simulink model "tankcontrol_linearised_model_PI_controller_control101"  (R2025b)
settings: Solver=VariableStepAuto  StartTime=0.0  StopTime=300  RelTol=1e-3
undefined symbols (not defined in the file or in its folder): alfa1rel, alfa2rel, beta1rel, delta2rel, h10rel, h20rel, u0
settings Model: Creator=barsr  LastModifiedBy=barsr
settings RTWCC: GPUComputeCapability=3.5

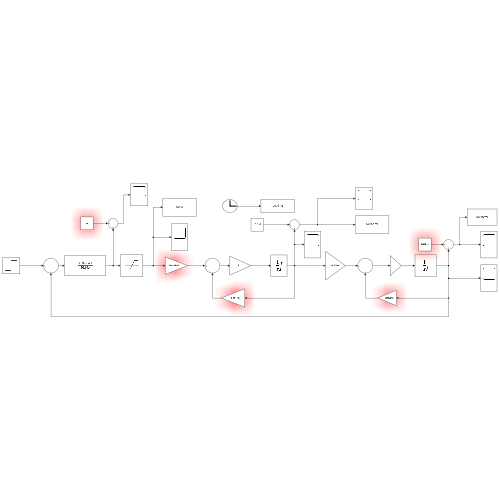
[thumbnail: Simulink's stored preview of the top-level diagram]
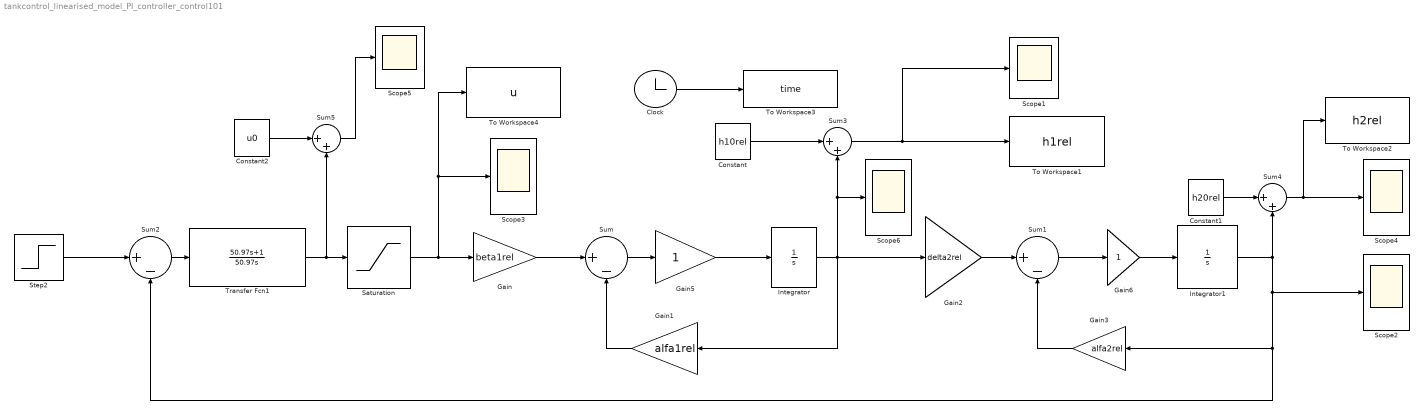
== system tankcontrol_linearised_model_PI_controller_control101 ==
  Clock : Clock
  Constant : Constant  Value=h10rel
  Constant1 : Constant  Value=h20rel
  Constant2 : Constant  Value=u0
  Gain : Gain  Gain=beta1rel
  Gain1 : Gain  Gain=alfa1rel
  Gain2 : Gain  Gain=delta2rel
  Gain3 : Gain  Gain=alfa2rel
  Gain5 : Gain
  Gain6 : Gain
  Integrator : Integrator  LimitOutput=on  UpperSaturationLimit=1  LowerSaturationLimit=0
  Integrator1 : Integrator  LimitOutput=on  UpperSaturationLimit=1  LowerSaturationLimit=0
  Saturation : Saturate  UpperLimit=1  LowerLimit=0
  Scope{1..6} (6 alike) : Scope
      Scope1 settings: ActiveDisplayYMinimum=0.047933990579917485  ActiveDisplayYMaximum=0.4377411736304716
      Scope2 settings: ActiveDisplayYMinimum=-0.76866162703230412  ActiveDisplayYMaximum=1.4291405570926656
      Scope3 settings: ActiveDisplayYMinimum=-0.82951581487383041  ActiveDisplayYMaximum=2.9648640057466338
      Scope4 settings: ActiveDisplayYMinimum=-0.76866162703230412  ActiveDisplayYMaximum=1.4291405570926656  DataLoggingVariableName=ScopeData2
      Scope5 settings: ActiveDisplayYMinimum=-0.28268319394776326  ActiveDisplayYMaximum=0.65543427021264211  DataLoggingVariableName=ScopeData3
      Scope6 settings: ActiveDisplayYMinimum=-0.76866162703230412  ActiveDisplayYMaximum=1.4291405570926656  DataLoggingVariableName=ScopeData4
  Step2 : Step  Time=0  After=0.3  SampleTime=0
  Sum : Sum  Inputs=|+-
  Sum1 : Sum  Inputs=|+-
  Sum2 : Sum  Inputs=|+-
  Sum3 : Sum  Inputs=|++
  Sum4 : Sum  Inputs=|++
  Sum5 : Sum  Inputs=|++
  To Workspace1 : ToWorkspace  VariableName=h1rel  SampleTime=-1
  To Workspace2 : ToWorkspace  VariableName=h2rel  SampleTime=-1
  To Workspace3 : ToWorkspace  VariableName=time  SampleTime=-1
  To Workspace4 : ToWorkspace  VariableName=u  SampleTime=-1
  Transfer Fcn1 : TransferFcn  Numerator=[50.97 1]  Denominator=[50.97 0]
  wires:
  Gain/1 -> Sum/1
  Sum/1 -> Gain5/1
  Integrator/1 -> Gain2/1, Gain1/1, Scope6/1, Sum3/2
  Sum1/1 -> Gain6/1
  Gain5/1 -> Integrator/1
  Gain6/1 -> Integrator1/1
  Gain1/1 -> Sum/2
  Gain3/1 -> Sum1/2
  Clock/1 -> To Workspace3/1
  Step2/1 -> Sum2/1
  Sum2/1 -> Transfer Fcn1/1
  Saturation/1 -> To Workspace4/1, Scope3/1, Gain/1
  Constant/1 -> Sum3/1
  Sum3/1 -> Scope1/1, To Workspace1/1
  Constant1/1 -> Sum4/1
  Gain2/1 -> Sum1/1
  Sum4/1 -> To Workspace2/1, Scope4/1
  Integrator1/1 -> Sum4/2, Scope2/1, Gain3/1, Sum2/2
  Transfer Fcn1/1 -> Saturation/1, Sum5/2
  Constant2/1 -> Sum5/1
  Sum5/1 -> Scope5/1
